simulink model "k1vists"  (Simulink 8.8)
settings: Solver=ode45  StartTime=0.0  StopTime=10.0  RelTol=1e-3  EnableMultiTasking=on
libraries: cdsFilt x9, cdsFunctionCall x2, cdsAdcx0 x1, cdsAdcx1 x1, rtdemod x1, cdsTP x1, cdsEpicsOut x1, cdsOsc x1, cdsParameters x1
settings Model: SuppressorTable=22 serialization::archive 11 0 3 0 0 0 11 0  Creator=keiko  LastModifiedBy=controls
settings DataIOCC: SignalLoggingSaveFormat=Dataset
settings DebuggingCC: UnderspecifiedInitializationDetection=Simplified  MergeDetectMultiDrivingBlocksExec=error  SolverPrmCheckMsg=warning  FcnCallInpInsideContextMsg=error  AllowSymbolicDim=off  StateNameClashWarn=none
settings GRTTargetCC: CombineOutputUpdateFcns=on  GRTInterface=off

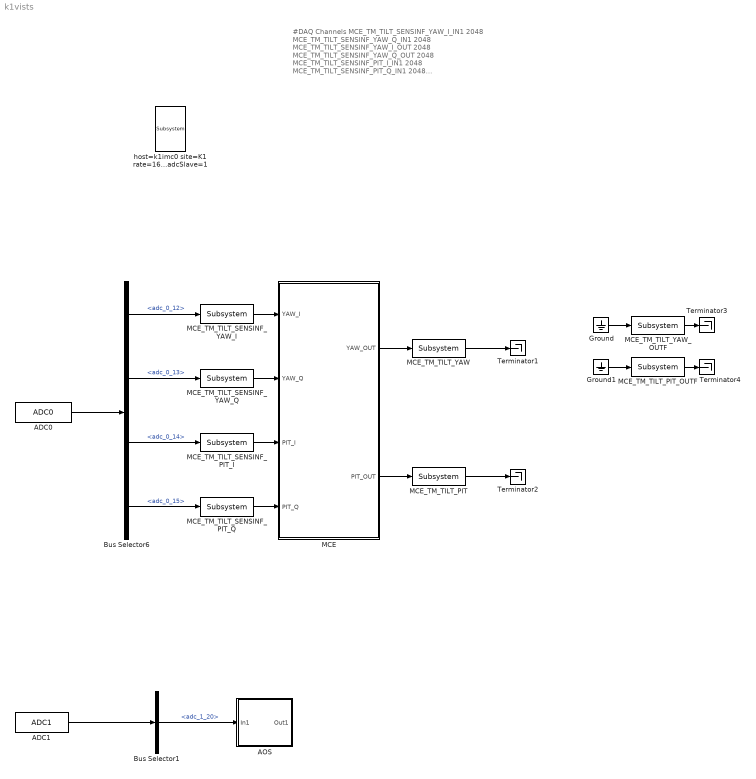
== system k1vists ==
  note: #DAQ Channels
      | MCE_TM_TILT_SENSINF_YAW_I_IN1 2048
      | MCE_TM_TILT_SENSINF_YAW_Q_IN1 2048
      | MCE_TM_TILT_SENSINF_YAW_I_OUT 2048
      | MCE_TM_TILT_SENSINF_YAW_Q_OUT 2048
      | MCE_TM_TILT_SENSINF_PIT_I_IN1 2048
      | MCE_TM_TILT_SENSINF_PIT_Q_IN1 2048
      | MCE_TM_TILT_SENSINF_PIT_I_OUT 2048
      | MCE_TM_TILT_SENSINF_PIT_Q_OUT 2048
      | MCE_TM_TILT_YAW_IN1 2048
      | MCE_TM_TILT_YAW_OUT 2048
      | MCE_TM_TILT_PIT_IN1 2048
      | MCE_TM_TILT_PIT_OUT 2048
      | MCE_TM_TILT_PIT_OUTF_OUT 2048
      | MCE_TM_TILT_YAW_OUTF_OUT 2048
      | AOS_HPBD_IFI_TEMPERATURE_OUT 2048
  ADC0 : cdsAdcx0/ADC0  Tag=cdsAdc  Description=|
      | type-GSC_16AI64SSA
      | card_num=0
      settings: AttributesFormatString=%<Description>\n%<Tag>
  ADC1 : cdsAdcx1/ADC1  Tag=cdsAdc  Description=|
      | type-GSC_16AI64SSA
      | card_num=1
      settings: AttributesFormatString=%<Description>\n%<Tag>
  AOS : Subsystem  Tag=top_names
  Bus Selector1 : BusSelector  Description=ADC Selector  OutputSignals=adc_1_20
      settings: AttributesFormatString=%<Description>
  Bus Selector6 : BusSelector  Description=ADC Selector  OutputSignals=adc_0_12,adc_0_13,adc_0_14,adc_0_15
      settings: AttributesFormatString=%<Description>
  Ground : Ground
  Ground1 : Ground
  MCE : Subsystem
  MCE_TM_TILT_PIT : cdsFilt/Subsystem  Tag=cdsFilt  Description=ADL=LOCKIN_FILTER.adl
      settings: AttributesFormatString=%<Tag>
  MCE_TM_TILT_PIT_OUTF : cdsFilt/Subsystem  Tag=cdsFilt  Description=ADL=LOCKIN_FILTER.adl
      settings: AttributesFormatString=%<Tag>
  MCE_TM_TILT_SENSINF_PIT_I : cdsFilt/Subsystem  Tag=cdsFilt  Description=ADL=LOCKIN_FILTER.adl
      settings: AttributesFormatString=%<Tag>
  MCE_TM_TILT_SENSINF_PIT_Q : cdsFilt/Subsystem  Tag=cdsFilt  Description=ADL=LOCKIN_FILTER.adl
      settings: AttributesFormatString=%<Tag>
  MCE_TM_TILT_SENSINF_YAW_I : cdsFilt/Subsystem  Tag=cdsFilt  Description=ADL=LOCKIN_FILTER.adl
      settings: AttributesFormatString=%<Tag>
  MCE_TM_TILT_SENSINF_YAW_Q : cdsFilt/Subsystem  Tag=cdsFilt  Description=ADL=LOCKIN_FILTER.adl
      settings: AttributesFormatString=%<Tag>
  MCE_TM_TILT_YAW : cdsFilt/Subsystem  Tag=cdsFilt  Description=ADL=LOCKIN_FILTER.adl
      settings: AttributesFormatString=%<Tag>
  MCE_TM_TILT_YAW_OUTF : cdsFilt/Subsystem  Tag=cdsFilt  Description=ADL=LOCKIN_FILTER.adl
      settings: AttributesFormatString=%<Tag>
  Terminator{1..4} (4 alike) : Terminator
  host=k1imc0 site=K1 rate=16K dcuid=41 specific_cpu=5 adcSlave=1 : cdsParameters/Subsystem  Tag=cdsParameters  Description=|
      | Purpose:                                                                                                                                                                                                                                
      | Provide system parameters to the FE code generator to properly configure the generated EPICS names, rep rate of the FE controller, and the Data Acquisition node ID for proper storage of data from this FE controller.                 
      |                                                                                                                                                                                                                                         
      | Useage:                                                                                                                                                                                                                                 
      | The part NAME field is used to identify the FE parameters. It must be of the form:                                                                                                                                                      
      | site=                                                                                                                                                                                                                                   
      | rate=                                                                                                                                                                                                                                   
      | dcuid=                                                                                                                                                                                                                                  
      |                                                                                                                                                                                                                                         
      | Where:                                                                                                                                                                                                                                  
      | site= argument may be H1, H2, L1, M1, G1, either as a single argument or multiple, for example site=H1,H2. These are the only names allowed. These will become the first two characters of all EPICS and signal names (for example G1:).
      |                                                                                                                                                                                                                                         
      | rate= may be 2K, 16K, 32K, or 64K                                                                                                                                                                                                       
      |                                                                                                                                                                                                                                         
      | dcuid= is site specific ie it must be unique at each site.
      settings: AttributesFormatString=%<Tag>
  wires:
  ADC0/1 -> Bus Selector6/1
  Bus Selector6/2 -> MCE_TM_TILT_SENSINF_YAW_Q/1  "<adc_0_13>"
  Bus Selector6/1 -> MCE_TM_TILT_SENSINF_YAW_I/1  "<adc_0_12>"
  Bus Selector6/3 -> MCE_TM_TILT_SENSINF_PIT_I/1  "<adc_0_14>"
  MCE/1(YAW_OUT) -> MCE_TM_TILT_YAW/1
  MCE/2(PIT_OUT) -> MCE_TM_TILT_PIT/1
  Bus Selector6/4 -> MCE_TM_TILT_SENSINF_PIT_Q/1  "<adc_0_15>"
  MCE_TM_TILT_SENSINF_YAW_I/1 -> MCE/1(YAW_I)
  MCE_TM_TILT_SENSINF_YAW_Q/1 -> MCE/2(YAW_Q)
  MCE_TM_TILT_SENSINF_PIT_I/1 -> MCE/3(PIT_I)
  MCE_TM_TILT_SENSINF_PIT_Q/1 -> MCE/4(PIT_Q)
  MCE_TM_TILT_YAW/1 -> Terminator1/1
  MCE_TM_TILT_PIT/1 -> Terminator2/1
  MCE_TM_TILT_YAW_OUTF/1 -> Terminator3/1
  MCE_TM_TILT_PIT_OUTF/1 -> Terminator4/1
  Ground/1 -> MCE_TM_TILT_YAW_OUTF/1
  Ground1/1 -> MCE_TM_TILT_PIT_OUTF/1
  ADC1/1 -> Bus Selector1/1
  Bus Selector1/1 -> AOS/1(In1)  "<adc_1_20>"

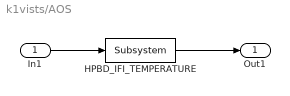
== system k1vists/AOS ==
  In1 : Inport
  HPBD_IFI_TEMPERATURE : cdsFilt/Subsystem  Tag=cdsFilt  Description=ADL=LOCKIN_FILTER.adl
      settings: AttributesFormatString=%<Tag>
  Out1 : Outport
  wires:
  HPBD_IFI_TEMPERATURE/1 -> Out1/1
  In1/1 -> HPBD_IFI_TEMPERATURE/1

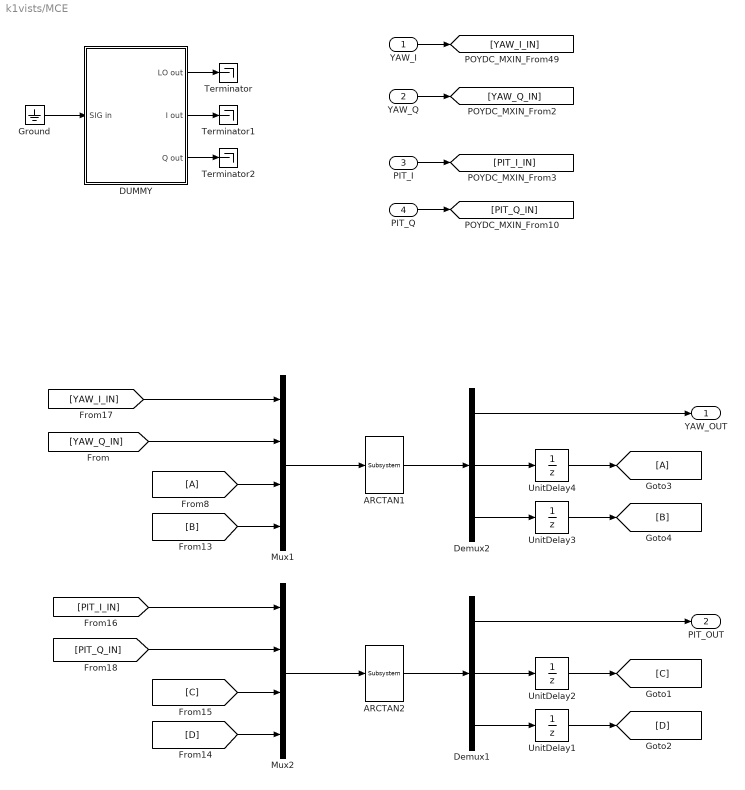
== system k1vists/MCE ==
  YAW_I : Inport
  YAW_Q : Inport  Port=2
  PIT_I : Inport  Port=3
  PIT_Q : Inport  Port=4
  ARCTAN1 : cdsFunctionCall/Subsystem  Tag=cdsFunctionCall  Description=inline ARCTAN /opt/rtcds/userapps/release/vis/common/src/ARCTAN.c
      settings: AttributesFormatString=%<Tag>\n%<Description>
  ARCTAN2 : cdsFunctionCall/Subsystem  Tag=cdsFunctionCall  Description=inline ARCTAN /opt/rtcds/userapps/release/vis/common/src/ARCTAN.c
      settings: AttributesFormatString=%<Tag>\n%<Description>
  DUMMY : Subsystem  Description=ADL=LOCKIN.adl
      settings: AttributesFormatString=%<Tag>
  Demux1 : Demux  Outputs=3
  Demux2 : Demux  Outputs=3
  Ground : Ground
  Mux1 : Mux
  Mux2 : Mux
  Terminator : Terminator
  Terminator1 : Terminator
  Terminator2 : Terminator
  UnitDelay{1..4} (4 alike) : UnitDelay
  YAW_OUT : Outport
  PIT_OUT : Outport  Port=2
  wires:
  UnitDelay4/1 -> [A]
  UnitDelay3/1 -> [B]
  UnitDelay2/1 -> [C]
  UnitDelay1/1 -> [D]
  [D] -> Mux2/4
  [C] -> Mux2/3
  Demux1/3 -> UnitDelay1/1
  Demux1/2 -> UnitDelay2/1
  ARCTAN2/1 -> Demux1/1
  Mux2/1 -> ARCTAN2/1
  [B] -> Mux1/4
  [A] -> Mux1/3
  Demux2/3 -> UnitDelay3/1
  Demux2/2 -> UnitDelay4/1
  ARCTAN1/1 -> Demux2/1
  Mux1/1 -> ARCTAN1/1
  Demux1/1 -> PIT_OUT/1
  PIT_I/1 -> [PIT_I_IN]
  Demux2/1 -> YAW_OUT/1
  YAW_Q/1 -> [YAW_Q_IN]
  PIT_Q/1 -> [PIT_Q_IN]
  [YAW_Q_IN] -> Mux1/2
  [PIT_I_IN] -> Mux2/1
  [PIT_Q_IN] -> Mux2/2
  [YAW_I_IN] -> Mux1/1
  YAW_I/1 -> [YAW_I_IN]
  DUMMY/1(LO out) -> Terminator/1
  DUMMY/2(I out) -> Terminator1/1
  DUMMY/3(Q out) -> Terminator2/1
  Ground/1 -> DUMMY/1(SIG in)

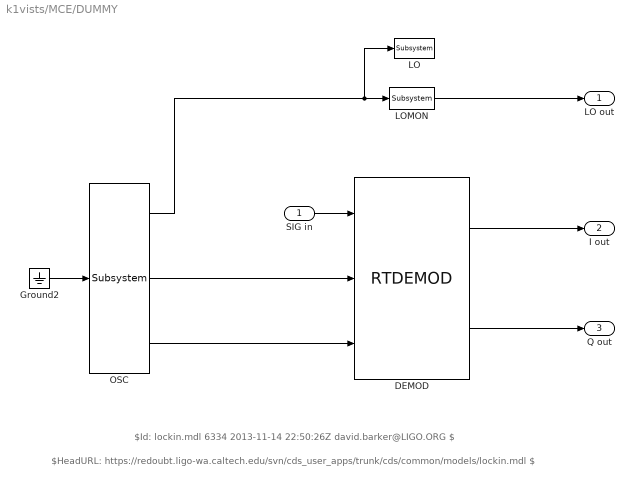
== system k1vists/MCE/DUMMY ==
  note: $Id: lockin.mdl 6334 2013-11-14 22:50:26Z david.barker@LIGO.ORG $
  note: $HeadURL: https://redoubt.ligo-wa.caltech.edu/svn/cds_user_apps/trunk/cds/common/models/lockin.mdl $
  SIG in : Inport
  DEMOD : rtdemod/RTDEMOD
  Ground2 : Ground
  LO : cdsTP/Subsystem  Tag=Test Point
      settings: AttributesFormatString=%<Tag>
  LOMON : cdsEpicsOut/Subsystem  Tag=cdsEpicsOutput  Description=|
      | Purpose:                                          
      | Output a FE signal to an EPICS channel.           
      |                                                   
      | Operation:                                        
      | Takes input value and passes it to EPICS record.  
      |                                                   
      | Usage:                                            
      | Name the part with the desired EPICS rrecord name.
      settings: AttributesFormatString=%<Tag>
  OSC : cdsOsc/Subsystem  Tag=cdsOsc  Description=Oscillator
      settings: AttributesFormatString=%<Tag>
  LO out : Outport
  I out : Outport  Port=2
  Q out : Outport  Port=3
  wires:
  OSC/1 -> LOMON/1, LO/1
  OSC/2 -> DEMOD/2
  OSC/3 -> DEMOD/3
  LOMON/1 -> LO out/1
  DEMOD/2 -> Q out/1
  DEMOD/1 -> I out/1
  SIG in/1 -> DEMOD/1
  Ground2/1 -> OSC/1
